simulink model "modele3"  (R2024a)
settings: Solver=VariableStepAuto  StartTime=0  StopTime=10  RelTol=1e-10
undefined symbols (not defined in the file or in its folder): A_L, A_S, C_x, calcul_adherence, calcul_delta, calcul_forceaero, calcul_forces, calcul_lambda, calcul_N, calcul_omega, calcul_retourvitesse, calcul_rotaroute, calcul_slipangle, calcul_vitessesroues, Cte_1, Cte_2, Cte_3, Cte_4, d_f, d_r, eqpfd, f, g, h, Iz, J, L, l_f, l_r, M, projection, R, rho
libraries: slpidlib x1, cstblocks x1
settings Model: Creator=TP-EEA  LastModifiedBy=TP-EEA
settings DebuggingCC: UnconnectedInputMsg=warning  UnconnectedOutputMsg=warning  UnconnectedLineMsg=warning
settings ModelReferenceCC: EnableRefExpFcnMdlSchedulingChecks=on
settings RTWCC: GPUComputeCapability=3.5  DLArmComputeVersion=19.05

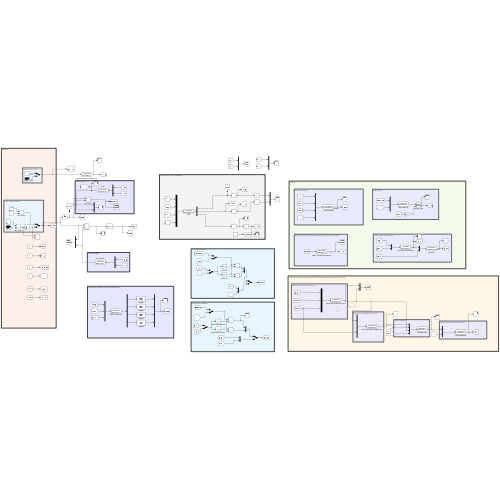
[thumbnail: Simulink's stored preview of the top-level diagram]
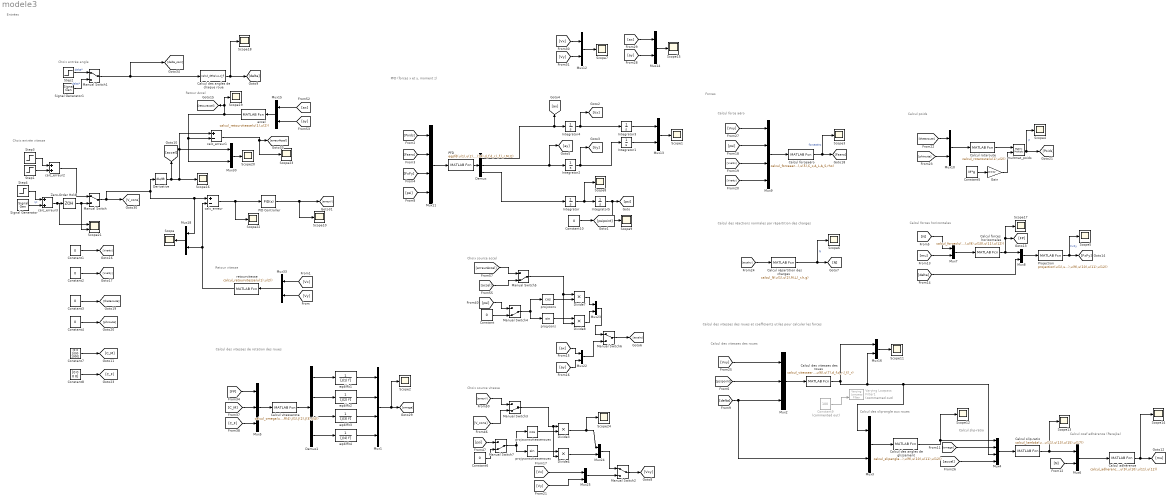
== system modele3 ==
  note: PFD (forces x et y, moment z)
  note: Forces
  note: Choix entrée vitesse
  note: Choix entrée angle
  note: Retour Accel
  note: Retour vitesse
  note: Entrées
  note: Calcul poids
  note: Calcul force aéro
  note: Calcul des réactions normales par répartition des charges
  note: Calcul slip-ratio
  note: Calcul coef adhérence (Pacejka)
  note: Calcul des slip-angle aux roues
  note: Calcul des vitesses des roues
  note: Calcul des vitesses des roues et coefficients utiles pour calculer les forces
  note: Calcul des vitesses de rotation des roues
  note: Calcul forces horizontales
  note: Choix source accel
  note: Choix source vitesse
  Calcul adhérence : MATLABFcn  MATLABFcn=calcul_adherence(u(1),u(2),u(3),u(4),u(5),u(6),u(7),u(8),Cte_1,Cte_2,Cte_3,Cte_4,u(9),u(10),u(11),u(12))  OutputDimensions=4*2
  Calcul des angles de chaque roue : MATLABFcn  MATLABFcn=calcul_delta(u,L,d_f)  OutputDimensions=4
  Calcul des angles de glissement : MATLABFcn  MATLABFcn=calcul_slipangle(u(1),u(2),u(3),u(4),u(5),u(6),u(7),u(8),u(9),u(10),u(11),u(12))  OutputDimensions=4
  Calcul des vitesses des roues : MATLABFcn  MATLABFcn=calcul_vitessesroues(u(1),u(2),u(3),u(4),u(5),u(6),u(7),d_f,d_r,l_f,l_r)  OutputDimensions=8
  Calcul forceaéro : MATLABFcn  MATLABFcn=calcul_forceaero(u(1),u(2),u(3),u(4),u(5),C_x,A_L,A_S,rho)  OutputDimensions=2
  Calcul forces horizontales : MATLABFcn  MATLABFcn=calcul_forces(u(1),u(2),u(3),u(4),u(5),u(6),u(7),u(8),u(9),u(10),u(11),u(12))  OutputDimensions=4*2
  Calcul rotaroute : MATLABFcn  MATLABFcn=calcul_rotaroute(u(1),u(2))  OutputDimensions=[3 3]  Output1D=off
  Calcul répartition des charges : MATLABFcn  MATLABFcn=calcul_N(u(1),u(2),M,L,l_r,h,g)  OutputDimensions=4
  Calcul slip-ratio : MATLABFcn  MATLABFcn=calcul_lambda(u(1),u(2),u(3),u(4),R(1),R(2),R(3),R(4),u(5),u(6),u(7),u(8),u(9),u(11),u(13),u(15),u(17))  OutputDimensions=4*2
  Calcul vitesserota : MATLABFcn  MATLABFcn=calcul_omega(u(1),u(2),u(3),u(4),u(5),u(6),u(7),u(8),u(9),u(10),u(11),u(12),u(13),u(14),u(15),u(16),R(1),R(2),R(3),R(4),J(1),J(2),J(3),J(4))  OutputDimensions=4
  Constant{,1..4,6,10} (7 alike) : Constant  Value=0
  Constant5 : Constant  Value=M*g  VectorParams1D=off
  Constant7 : Constant  Value=[0 0 1000 1000]
  Constant8 : Constant  Value=[0 0 0 0]
  Constant9 : Constant  Commented=on  Value=100
  Demux : Demux  Outputs=3
  Demux1 : Demux
  Derivative : Derivative
  Divide{3..4,7..8} (4 alike) : Product  Inputs=**
  Gain : Gain  Gain=[0 0 1]'
  Integrator{,1..5} (6 alike) : Integrator
  Manual Switch{,1..2,6} (4 alike) : ManualSwitch
  Manual Switch{3..5,7} (4 alike) : ManualSwitch  CurrentSetting=0
  Mux{1,4,9,11} (4 alike) : Mux
  Mux{3,6..8,10,12..16,18,22..25,30,33} (17 alike) : Mux  Inputs=2
  Mux2 : Mux  Inputs=3
  Mux5 : Mux  Inputs=3
  PFD : MATLABFcn  MATLABFcn=eqpfd(u(1),u(2),u(4),u(5),u(6),u(7),u(8),u(9),u(10),u(11),u(12),u(13),u(14),d_f,d_r,l_f,l_r,M,Iz)  OutputDimensions=3
  PID Controller : slpidlib/PID Controller  Controller=PID  Form=Parallel  TimeDomain=Continuous-time  UseExternalTs=off  SampleTime=-1  IntegratorMethod=Forward Euler  FilterMethod=Forward Euler  ControllerParametersSource=internal  P=1  I=1  UseKiTs=off  D=0  UseExternalDerivativeSource=off  N=5000  UseFilter=on  TunerSelectOption=Frequency Response Based  InitialConditionSource=internal  InitialConditionForIntegrator=0  InitialConditionForFilter=0  DifferentiatorICPrevScaledInput=0  ExternalReset=none  TrackingMode=off  Kt=1  LimitOutput=off  SatLimitsSource=internal  UpperSaturationLimit=inf  LowerSaturationLimit=-inf  LinearizeAsGain=on  AntiWindupMode=none  Kb=1  LimitIntegrator=off  UpperIntegratorSaturationLimit=inf  LowerIntegratorSaturationLimit=-inf  POutMin=[]  POutMax=[]  IOutMin=[]  IOutMax=[]  DOutMin=[]  DOutMax=[]  NOutMin=[]  NOutMax=[]  SumOutMin=[]  SumOutMax=[]  SaturationOutMin=[]  SaturationOutMax=[]  PParamMin=[]  PParamMax=[]  IParamMin=[]  IParamMax=[]  DParamMin=[]  DParamMax=[]  NParamMin=[]  NParamMax=[]  KbParamMin=[]  KbParamMax=[]  KtParamMin=[]  KtParamMax=[]  KbOutMin=[]  KbOutMax=[]  KtOutMin=[]  KtOutMax=[]  IntegratorOutMin=[]  IntegratorOutMax=[]  FilterOutMin=[]  FilterOutMax=[]  SumI1OutMin=[]  SumI1OutMax=[]  SumI2OutMin=[]  SumI2OutMax=[]  SumI3OutMin=[]  SumI3OutMax=[]  SumI4OutMin=[]  SumI4OutMax=[]  SumDOutMin=[]  SumDOutMax=[]  DifferentiatorOutMin=[]  DifferentiatorOutMax=[]  FilterDiffOutCoefMin=[]  FilterDiffOutCoefMax=[]  ReciprocalOutMin=[]  ReciprocalOutMax=[]  SumDenOutMin=[]  SumDenOutMax=[]  SumNumOutMin=[]  SumNumOutMax=[]  DivideOutMin=[]  DivideOutMax=[]  UdiffTsProdOutMin=[]  UdiffTsProdOutMax=[]  NTsProdOutMin=[]  NTsProdOutMax=[]  UintegralTsProdOutMin=[]  UintegralTsProdOutMax=[]  UngainTsProdOutMin=[]  UngainTsProdOutMax=[]  ClampingZeroOutDataTypeStr=Inherit: Inherit via back propagation  ClampingZeroOutMin=[]  ClampingZeroOutMax=[]  FilterDenConstantOutDataTypeStr=Inherit: Inherit via back propagation  FilterDenConstantOutMin=[]  FilterDenConstantOutMax=[]  PCopyOutDataTypeStr=Inherit: Inherit via back propagation  PCopyOutMin=[]  PCopyOutMax=[]  NCopyOutDataTypeStr=Inherit: Inherit via back propagation  NCopyOutMin=[]  NCopyOutMax=[]  IntegratorContinuousStateAttributes=''  IntegratorStateMustResolveToSignalObject=off  IntegratorRTWStateStorageClass=Auto  FilterContinuousStateAttributes=''  FilterStateMustResolveToSignalObject=off  FilterRTWStateStorageClass=Auto  ParallelPVariant=InternalParameters  IdealPVariant=Disabled  IVariant=InternalParameters  DVariant=InternalParameters  IntegratorVariant=Continuous  SatVariant=Disabled  AWVariant=Passthrough  PCopyVariant=Disabled  TRVariant=Disabled  FdbkBlocksVariant=Forward  IdealPFdbkVariant=Disabled  SatFdbkVariant=Disabled  DerivativeFilterVariant=ContFilter  NVariant=InternalParameters  NCopyVariant=Disabled  FilterICVariant=InternalICsFilter  IntegratorICVariant=InternalICs  ExternalResetVariant=Disabled  TRSumVariant=Passthrough  SumFdbkVariant=Disabled  SumVariant=Sum_PID  TsampFilterVariant=InternalTs  TsampNgainVariant=Passthrough  TsampIntegralVariant=Disabled_SignalSpec  ExternalSaturationOutDataTypeStr=Inherit: Same as second input  DerivativeSourceVariant=ErrorSignal
  Projection : MATLABFcn  MATLABFcn=projection(u(1),u(2),u(3),u(4),u(5),u(6),u(7),u(8),u(9),u(10),u(11),u(12))  OutputDimensions=8
  Scope{,1..20,22..24} (24 alike) : Scope
  Scope21 : Scope  NumInputPorts=2
  Signal Generator : SignalGenerator  Amplitude=10/3.6  Frequency=0.05
  Signal Generator1 : SignalGenerator  Frequency=0.01  Units=rad/sec
  Step1 : Step  Time=0  After=10/3.6  SampleTime=0
  Step2 : Step  Time=0  After=0  SampleTime=0
  Step3 : Step  Time=5  After=0  SampleTime=0
  Step4 : Step  Time=0  After=20/3.6  SampleTime=0
  Varying Lowpass Filter1 : cstblocks/Linear Parameter Varying/Varying Lowpass Filter  Commented=on  N=5
  Zero-Order Hold : ZeroOrderHold  SampleTime=0.5
  accel : MATLABFcn  MATLABFcn=calcul_retourvitesse(u(1),u(2))  OutputDimensions=1
  calc_erreur : Sum  Inputs=+-
  calc_erreur1 : Sum  Inputs=+-
  calc_erreur2 : Sum
  calc_erreur3 : Sum
  eqdiffz1 : TransferFcn  Denominator=[J(1) f]
  eqdiffz2 : TransferFcn  Denominator=[J(2) f]
  eqdiffz3 : TransferFcn  Denominator=[J(3) f]
  eqdiffz4 : TransferFcn  Denominator=[J(4) f]
  multmat_poids : Product  Multiplication=Matrix(*)
  projxcons : Trigonometry  Operator=cos
  projxconsvitesseroues : Trigonometry  Operator=cos
  projycons : Trigonometry
  projyconsvitesseroues : Trigonometry
  retourvitesse : MATLABFcn  MATLABFcn=calcul_retourvitesse(u(1),u(2))  OutputDimensions=1
  wires:
  calc_erreur1/1 -> [erreurAccel], Scope23/1
  Constant1/1 -> [Vventx]
  Manual Switch1/1 -> [delta_com], Calcul des angles de chaque roue/1
  Manual Switch/1 -> calc_erreur/1, Mux18/1, Derivative/1, [V_cons]
  Mux30/1 -> Scope20/1
  Mux18/1 -> Scope/1
  [ay] -> Mux15/2
  Step2/1 -> Manual Switch1/1  "delta*"
  Signal Generator1/1 -> Manual Switch1/2  "delta*"
  [ax] -> Mux15/1
  Derivative/1 -> Scope16/1, Mux30/1, calc_erreur1/1, [accel]
  Constant8/1 -> [C_F]
  Constant7/1 -> [C_M]
  Constant3/1 -> [thetaroute]
  retourvitesse/1 -> calc_erreur/2, Mux18/2
  Constant4/1 -> [phiroute]
  Calcul des angles de chaque roue/1 -> [delta], Scope18/1
  [Vx] -> Mux33/1
  [Vy] -> Mux33/2
  Mux33/1 -> retourvitesse/1
  Constant2/1 -> [Vventy]
  Gain/1 -> multmat_poids/2
  Mux10/1 -> Calcul rotaroute/1
  multmat_poids/1 -> Scope4/1, [Poids]  "P"
  Constant5/1 -> Gain/1
  Calcul rotaroute/1 -> multmat_poids/1
  [phiroute] -> Mux10/2
  [thetaroute] -> Mux10/1
  [Vventy] -> Mux9/4
  Calcul forceaéro/1 -> Scope3/1, [Faero]  "forceaéro"
  [psi] -> Mux9/2
  [Vventx] -> Mux9/3
  Mux9/1 -> Calcul forceaéro/1
  Calcul répartition des charges/1 -> Scope6/1, [N]  "N"
  [N] -> Mux6/2
  [accel] -> Mux4/4
  [Vxy] -> Mux2/1
  [omega] -> Mux4/2
  Calcul slip-ratio/1 -> Scope13/1, Mux6/1
  Calcul adhérence/1 -> Scope14/1, [mu]
  Mux3/1 -> Calcul des angles de glissement/1
  Mux6/1 -> Calcul adhérence/1
  Calcul des angles de glissement/1 -> Scope12/1, Mux4/1
  [delta] -> Mux3/2, Mux2/3
  Mux2/1 -> Calcul des vitesses des roues/1
  [psipoint] -> Mux2/2
  Mux4/1 -> Calcul slip-ratio/1
  Mux1/1 -> Scope2/1, [omega]
  Mux5/1 -> Calcul vitesserota/1
  [C_F] -> Mux5/3
  Calcul vitesserota/1 -> Demux1/1
  [FP] -> Mux5/1
  [C_M] -> Mux5/2
  [delta] -> Mux8/2
  [N] -> Mux7/1
  Mux7/1 -> Calcul forces horizontales/1
  Mux8/1 -> Projection/1
  Projection/1 -> Scope5/1, [FxFy]  "FxFy"
  Calcul forces horizontales/1 -> Scope17/1, [FP], Mux8/1
  [mu] -> Mux7/2
  Integrator5/1 -> Scope9/1, [psi]
  Integrator/1 -> Scope8/1, Integrator5/1
  [FxFy] -> Mux11/3
  [Faero] -> Mux11/2
  [Poids] -> Mux11/1
  [psi] -> Mux11/4
  Mux11/1 -> PFD/1
  PFD/1 -> Demux/1
  Integrator2/1 -> Integrator1/1, [Vy]
  Integrator4/1 -> [Vx], Integrator3/1
  Integrator3/1 -> Mux13/1
  Integrator1/1 -> Mux13/2
  Mux12/1 -> Scope7/1
  Mux13/1 -> Scope1/1
  Divide8/1 -> Mux23/2
  Divide3/1 -> Scope24/1, Mux24/1
  Mux24/1 -> Manual Switch2/1
  [ax] -> Mux22/1
  Mux22/1 -> Manual Switch6/2
  Mux23/1 -> Manual Switch6/1
  Divide7/1 -> Mux23/1
  Mux25/1 -> Manual Switch2/2
  [erreurV] -> Manual Switch3/1
  Divide4/1 -> Mux24/2
  projyconsvitesseroues/1 -> Divide4/1
  projxconsvitesseroues/1 -> Divide3/2
  projxcons/1 -> Divide7/2
  Manual Switch5/1 -> Divide8/2, Divide7/1
  [accel] -> Manual Switch5/2
  Manual Switch3/1 -> Divide4/2, Divide3/1
  [ay] -> Mux22/2
  [V_cons] -> Manual Switch3/2
  Manual Switch6/1 -> [accelxy]
  projycons/1 -> Divide8/1
  [Vy] -> Mux25/2
  [erreurAccel] -> Manual Switch5/1
  [Vx] -> Mux25/1
  Manual Switch2/1 -> [Vxy]
  [Vxy] -> Mux9/1
  eqdiffz1/1 -> Mux1/1
  eqdiffz4/1 -> Mux1/4
  eqdiffz3/1 -> Mux1/3
  eqdiffz2/1 -> Mux1/2
  Demux1/4 -> eqdiffz4/1
  Demux1/1 -> eqdiffz1/1
  Demux1/2 -> eqdiffz2/1
  Demux1/3 -> eqdiffz3/1
  Mux14/1 -> Scope15/1
  Step1/1 -> calc_erreur2/2
  Step3/1 -> calc_erreur2/1
  calc_erreur2/1 -> Manual Switch/1
  [ax] -> Mux14/1
  [ay] -> Mux14/2
  [Vx] -> Mux12/1
  [Vy] -> Mux12/2
  Demux/3 -> Integrator/1
  calc_erreur/1 -> PID Controller/1, Scope22/1
  Manual Switch4/1 -> projycons/1, projxcons/1
  [psi] -> Manual Switch4/1
  Constant/1 -> Manual Switch4/2
  Manual Switch7/1 -> projxconsvitesseroues/1, projyconsvitesseroues/1
  [psi] -> Manual Switch7/1
  Constant6/1 -> Manual Switch7/2
  Zero-Order Hold/1 -> Scope21/2, Manual Switch/2
  accel/1 -> Mux30/2, calc_erreur1/2, Scope19/1, [retouraccel]
  Mux15/1 -> accel/1
  [accelxy] -> Calcul répartition des charges/1
  calc_erreur3/1 -> Scope21/1, Zero-Order Hold/1
  Signal Generator/1 -> calc_erreur3/2  "V*"
  Step4/1 -> calc_erreur3/1
  Demux/1 -> [ax], Integrator4/1
  Demux/2 -> Integrator2/1, [ay]
  Calcul des vitesses des roues/1 -> Mux16/2, Mux4/3, Mux3/1, Mux16/1
  Constant9/1 -> Varying Lowpass Filter1/2
  Mux16/1 -> Scope11/1
  PID Controller/1 -> Scope10/1, [erreurV]
  Constant10/1 -> [psipoint]
